simulink model "arch_logical"  (R2024a)
settings: Solver=ode23t  StartTime=0.0  StopTime=10.0  RelTol=1e-3
undefined symbols (not defined in the file): MCU_Ts, Param_SigProcessing_SpeedMeas_Delays, Req_Caps_Motor_Currents, Req_Caps_Motor_Torques, Req_Caps_Motor_Velocity, Req_Caps_Transmission_Torques, Req_Caps_Transmission_Velocity
libraries: simulink x5, mcbpositiondecoderlib x1
(part 2 of 2)

== system arch_logical/Sensing/Impairments ==
  Measurements In : Inport  OutDataTypeStr=Bus: Data_Measurements
  Ideal : Subsystem  VariantControl=Selector_Impairments == Types_Impairments.Ideal
      settings: PortSchema="{\"entries\":[{\"content\":{\"headerSize\":26,\"margin\":15,\"minimumSpacing\":25,\"sides\":[{\"content\":{\"connectorIds\":[\"Out1\"]},\"type\":\"ConnectorPlacement.EquallySpacedRectSide\",\"uuid\":\"adb94743-de46-43b3-8f5b-4e3d902d46b9\"},{\"content\":{\"connectorIds\":[\"In1\"],\"side\":\"RIGHT\"},\"type\":\"ConnectorPlacement.EquallySpacedRectSide\",\"uuid\":\"3d40f326-48c5-47c9-b6f5-5e68818bd70e\"},{\"content\":{\"side\":\"TOP\"},\"type\":\"ConnectorPlacement.EquallySpacedRectSide\",\"uuid\":\"35996a1f-7231-45c6-9398-88da53b9d412\"}]},\"type\":\"ConnectorPlacement.EquallySpacedConnector\",\"uuid\":\"901aa676-84bd-40f0-a38d-8b9c20d85e30\"}],\"packageUris\":[\"http://schema.mathworks.com/mf0/Connector/R2020b\"],\"version\":\"1.0\"}"
  Mk3 Serial Impairments : Subsystem  VariantControl=Selector_Impairments == Types_Impairments.Mk3_Serial  ReferencedSubsystem=Mk3SerialImpairments
      settings: PermitHierarchicalResolution=None  PortSchema="{\"entries\":[{\"content\":{\"headerSize\":26,\"margin\":15,\"minimumSpacing\":25,\"sides\":[{\"content\":{\"connectorIds\":[\"Out1\"]},\"type\":\"ConnectorPlacement.EquallySpacedRectSide\",\"uuid\":\"49c15c88-294a-49d3-a3e9-7e9d2d7e0fbb\"},{\"content\":{\"connectorIds\":[\"In1\"],\"side\":\"RIGHT\"},\"type\":\"ConnectorPlacement.EquallySpacedRectSide\",\"uuid\":\"231f3a62-e970-4c5e-be8a-7dda6d603d83\"},{\"content\":{\"side\":\"TOP\"},\"type\":\"ConnectorPlacement.EquallySpacedRectSide\",\"uuid\":\"403ac151-60ed-4891-8e31-1a38c9d325e1\"}]},\"type\":\"ConnectorPlacement.EquallySpacedConnector\",\"uuid\":\"3d0f34fd-30d8-4e40-9b1c-23769127a566\"}],\"packageUris\":[\"http://schema.mathworks.com/mf0/Connector/R2020b\"],\"version\":\"1.0\"}"
  Measurements Out : Outport  OutDataTypeStr=Bus: Data_Measurements

== system arch_logical/MCU/Planner/Planner None ==
  Bus Element In1 : Inport  PortName=Joint References In
  Bus Element Out1 : Outport  PortName=Joint References Out
  wires:
  Bus Element In1/1 -> Bus Element Out1/1

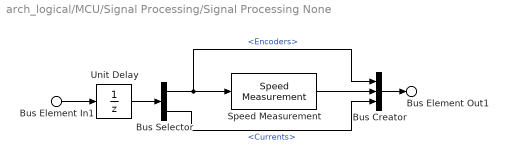
== system arch_logical/MCU/Signal Processing/Signal Processing None ==
  Bus Element In1 : Inport  PortName=Measurements
  Bus Creator : BusCreator  Inputs=3  OutDataTypeStr=Bus: Data_ControlFeedback  NonVirtualBus=on
      settings: InheritFromInputs=off
  Bus Selector : BusSelector  OutputSignals=Encoders,Currents
  Speed Measurement : mcbpositiondecoderlib/Speed Measurement  PositionUnit=Degrees  PositionScalingDatatype=uint32  SpeedCalculationMode=Time interval for speed calculation  SampleTimeAsync=MCU_Ts  MaximumApplicationSpeed=1000  SpeedResolution=10^-5/6  DelayLength=Param_SigProcessing_SpeedMeas_Delays  MaximumMeasurableSpeed=7499  MeasurableSpeedResolution=3.4925e-06  SpeedUnit=Degrees/Sec  PerUnitSpeed=1000  SpeedDataType=single
      settings: LibrarySourceBlock=mcblib/Sensor Decoders/Speed Measurement
  Unit Delay : UnitDelay  SampleTime=MCU_Ts  HasFrameUpgradeWarning=on
  Bus Element Out1 : Outport  PortName=Control Feedback
  wires:
  Bus Element In1/1 -> Unit Delay/1
  Unit Delay/1 -> Bus Selector/1
  Bus Creator/1 -> Bus Element Out1/1
  Bus Selector/1 -> Speed Measurement/1, Bus Creator/1  "<Encoders>"
  Bus Selector/2 -> Bus Creator/3  "<Currents>"
  Speed Measurement/1 -> Bus Creator/2

== system arch_logical/Sensing/Impairments/Ideal ==
  Bus Element In2 : Inport  PortName=Measurements In
  Bus Element Out1 : Outport  PortName=Measurements Out
  wires:
  Bus Element In2/1 -> Bus Element Out1/1
